simulink model "FIN_CARRERA_CARRO"  (R2023a)
settings: Solver=VariableStepAuto  StartTime=0.0  StopTime=10.0  RelTol=1e-3
settings Model: Creator=Ignacio  LastModifiedBy=Ignacio

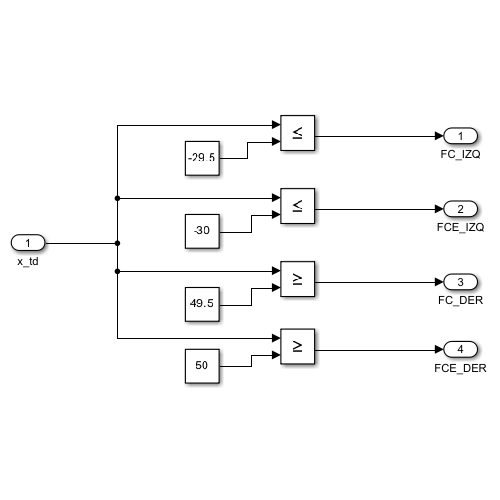
[thumbnail: Simulink's stored preview of the top-level diagram]
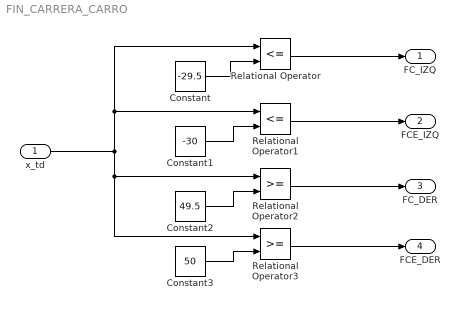
== system FIN_CARRERA_CARRO ==
  x_td : Inport
  Constant : Constant  Value=-29.5
  Constant1 : Constant  Value=-30
  Constant2 : Constant  Value=49.5
  Constant3 : Constant  Value=50
  Relational Operator : RelationalOperator  Operator=<=  OutDataTypeStr=boolean  RndMeth=Simplest  InputSameDT=off
  Relational Operator1 : RelationalOperator  Operator=<=  OutDataTypeStr=boolean  RndMeth=Simplest  InputSameDT=off
  Relational Operator2 : RelationalOperator  OutDataTypeStr=boolean  RndMeth=Simplest  InputSameDT=off
  Relational Operator3 : RelationalOperator  OutDataTypeStr=boolean  RndMeth=Simplest  InputSameDT=off
  FC_IZQ : Outport
  FCE_IZQ : Outport  Port=2
  FC_DER : Outport  Port=3
  FCE_DER : Outport  Port=4
  wires:
  x_td/1 -> Relational Operator3/1, Relational Operator2/1, Relational Operator/1, Relational Operator1/1
  Constant/1 -> Relational Operator/2
  Relational Operator/1 -> FC_IZQ/1
  Constant1/1 -> Relational Operator1/2
  Relational Operator1/1 -> FCE_IZQ/1
  Constant2/1 -> Relational Operator2/2
  Relational Operator2/1 -> FC_DER/1
  Constant3/1 -> Relational Operator3/2
  Relational Operator3/1 -> FCE_DER/1
